simulink model "PeakDetect"  (R2018b)
settings: Solver=FixedStepAuto  StartTime=1  StopTime=20  FixedStep=1  RelTol=1e-3
libraries: hdlsllib x4, simulink x2
settings Model: FPTRunName=FPA_Reference  Creator=jason  LastModifiedBy=jason
settings OptimizationCC: DefaultParameterBehavior=Inlined

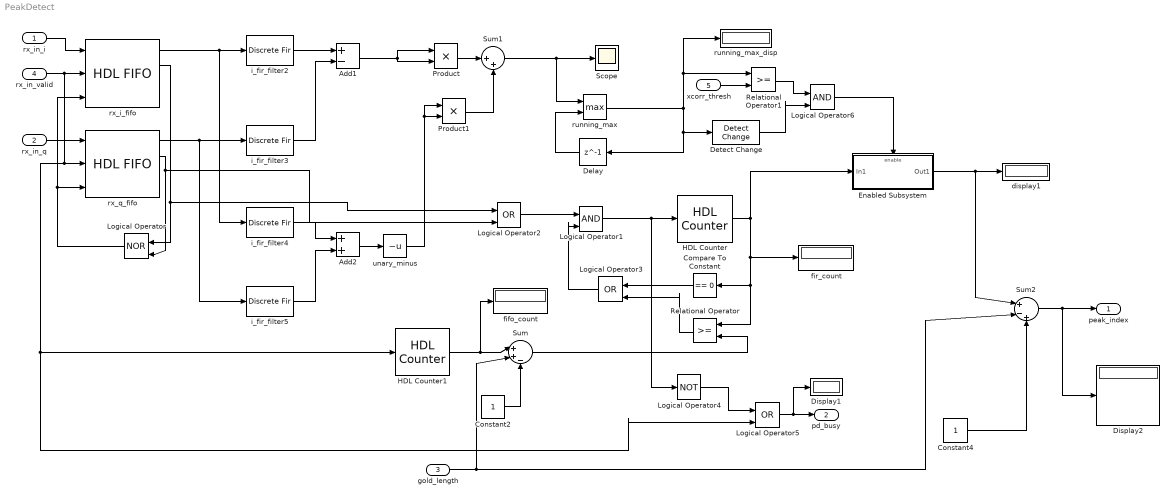
== system PeakDetect ==
  rx_in_i : Inport  OutDataTypeStr=fixdt(1,16,15)  SampleTime=1  Interpolate=off
  rx_in_q : Inport  Port=2  OutDataTypeStr=fixdt(1,16,15)  SampleTime=1  Interpolate=off
  gold_length : Inport  Port=3  OutDataTypeStr=uint16  Interpolate=off
  rx_in_valid : Inport  Port=4  OutDataTypeStr=boolean  SampleTime=1  Interpolate=off
  xcorr_thresh : Inport  Port=5  Interpolate=off
  Add1 : Sum  Inputs=+-
  Add2 : Sum
  Compare To Constant : simulink/Logic and Bit Operations/Compare To Constant  relop===  const=0  OutDataTypeStr=boolean
  Constant2 : Constant  OutDataTypeStr=uint8  SampleTime=-1
  Constant4 : Constant  OutDataTypeStr=uint16  SampleTime=-1
  Delay : Delay  DelayLength=1
  Detect Change : simulink/Logic and Bit Operations/Detect Change  vinit=0  OutDataTypeStr=boolean
  Display1 : Display
  Display2 : Display
  Enabled Subsystem : Subsystem  TreatAsAtomicUnit=on
  HDL Counter : hdlsllib/Sources/HDL Counter  CountType=Free running  CountInit=0  CountStep=1  CountMax=25  CountFromType=Initial value  CountFrom=0  CountResetPort=on  CountLoadPort=off  CountEnbPort=off  CountDirPort=off  CountDataType=Unsigned  CountWordLen=16  CountFracLen=0  CountSampTime=1
      settings: SourceProductBaseCode=HD
  HDL Counter1 : hdlsllib/Sources/HDL Counter  CountType=Free running  CountInit=0  CountStep=1  CountMax=25  CountFromType=Initial value  CountFrom=0  CountResetPort=off  CountLoadPort=off  CountEnbPort=on  CountDirPort=off  CountDataType=Unsigned  CountWordLen=16  CountFracLen=0  CountSampTime=1
      settings: SourceProductBaseCode=HD
  Logical Operator : Logic  Operator=NOR  IconShape=distinctive  AllPortsSameDT=off  OutDataTypeStr=boolean
  Logical Operator1 : Logic  IconShape=distinctive  AllPortsSameDT=off  OutDataTypeStr=boolean
  Logical Operator2 : Logic  Operator=OR  IconShape=distinctive  AllPortsSameDT=off  OutDataTypeStr=boolean
  Logical Operator3 : Logic  Operator=OR  IconShape=distinctive  AllPortsSameDT=off  OutDataTypeStr=boolean
  Logical Operator4 : Logic  Operator=NOT  IconShape=distinctive  AllPortsSameDT=off  OutDataTypeStr=boolean
  Logical Operator5 : Logic  Operator=OR  IconShape=distinctive  AllPortsSameDT=off  OutDataTypeStr=boolean
  Logical Operator6 : Logic  IconShape=distinctive  AllPortsSameDT=off  OutDataTypeStr=boolean
  Product : Product  OutDataTypeStr=Inherit: Inherit via back propagation
  Product1 : Product  OutDataTypeStr=Inherit: Inherit via back propagation
  Relational Operator : RelationalOperator  OutDataTypeStr=boolean  RndMeth=Nearest
  Relational Operator1 : RelationalOperator  OutDataTypeStr=boolean  RndMeth=Nearest
  Scope : Scope
  Sum : Sum  Inputs=|++-  AccumDataTypeStr=uint16
  Sum1 : Sum  Inputs=|++
  Sum2 : Sum  Inputs=|+-+  AccumDataTypeStr=uint16
  display1 : Display
  fifo_count : Display
  fir_count : Display
  i_fir_filter2 : DiscreteFir  Coefficients=fliplr([0.1538; 0.2282; 0.2753; 0.2904; 0.2678; 0.2226; 0.1475; 0.0555; -0.0424; -0.1347; -0.2101; -0.2594; -0.2722; -0.2594; -0.2101; -0.1347; -0.0424; 0.0555; 0.1475; 0.2226; 0.2763; 0.2977; 0.2794; 0.2276; 0.1477; 0.0478; -0.0623; -0.1725; -0.2689; -0.3564; -0.4163; -0.4493; -0.4546; -0.4329; -0.3872; -0.3214; -0.2364; -0.1508; -0.0581; 0.0313; 0.1114; 0.1768; 0.2233; 0.2478; 0.2445; 0.2267; 0.1835; 0.1230; 0.0499; -0.0298; -0.1101; -0.1852; -0.2545; -0.3086; -0.3404; -0.3536; -0.3500; -0.3325; -0.3055; -0.2736; -0.2459; -0.2136; -0.1926; -0.1807; -0.1788; -0.1865; -0.2027; -0.2254; -0.2478; -0.2799; -0.3056; -0.3262; -0.3387; -0.3401; -0.3282; -0.3015; -0.2637; -0.2106; -0.1396; -0.0592; 0.0251; 0.1067; 0.1795; 0.2379; 0.2826; 0.3069; 0.3069; 0.2909; 0.2651; 0.2369; 0.2138; 0.2018; 0.2005; 0.2156; 0.2494; 0.2914; 0.3326; 0.3631; 0.3737; 0.3572]')  ProductDataTypeStr=fixdt(1,64,32)  AccumDataTypeStr=fixdt(1,64,32)  OutDataTypeStr=fixdt(1,64,32)
  i_fir_filter3 : DiscreteFir  Coefficients=-1*fliplr([0.1538; 0.2282; 0.2753; 0.2904; 0.2678; 0.2226; 0.1475; 0.0555; -0.0424; -0.1347; -0.2101; -0.2594; -0.2722; -0.2594; -0.2101; -0.1347; -0.0424; 0.0555; 0.1475; 0.2226; 0.2763; 0.2977; 0.2794; 0.2276; 0.1477; 0.0478; -0.0623; -0.1725; -0.2689; -0.3564; -0.4163; -0.4493; -0.4546; -0.4329; -0.3872; -0.3214; -0.2364; -0.1508; -0.0581; 0.0313; 0.1114; 0.1768; 0.2233; 0.2478; 0.2445; 0.2267; 0.1835; 0.1230; 0.0499; -0.0298; -0.1101; -0.1852; -0.2545; -0.3086; -0.3404; -0.3536; -0.3500; -0.3325; -0.3055; -0.2736; -0.2459; -0.2136; -0.1926; -0.1807; -0.1788; -0.1865; -0.2027; -0.2254; -0.2478; -0.2799; -0.3056; -0.3262; -0.3387; -0.3401; -0.3282; -0.3015; -0.2637; -0.2106; -0.1396; -0.0592; 0.0251; 0.1067; 0.1795; 0.2379; 0.2826; 0.3069; 0.3069; 0.2909; 0.2651; 0.2369; 0.2138; 0.2018; 0.2005; 0.2156; 0.2494; 0.2914; 0.3326; 0.3631; 0.3737; 0.3572]')  ProductDataTypeStr=fixdt(1,64,32)  AccumDataTypeStr=fixdt(1,64,32)  OutDataTypeStr=fixdt(1,64,32)
  i_fir_filter4 : DiscreteFir  Coefficients=-1*fliplr([0.1538; 0.2282; 0.2753; 0.2904; 0.2678; 0.2226; 0.1475; 0.0555; -0.0424; -0.1347; -0.2101; -0.2594; -0.2722; -0.2594; -0.2101; -0.1347; -0.0424; 0.0555; 0.1475; 0.2226; 0.2763; 0.2977; 0.2794; 0.2276; 0.1477; 0.0478; -0.0623; -0.1725; -0.2689; -0.3564; -0.4163; -0.4493; -0.4546; -0.4329; -0.3872; -0.3214; -0.2364; -0.1508; -0.0581; 0.0313; 0.1114; 0.1768; 0.2233; 0.2478; 0.2445; 0.2267; 0.1835; 0.1230; 0.0499; -0.0298; -0.1101; -0.1852; -0.2545; -0.3086; -0.3404; -0.3536; -0.3500; -0.3325; -0.3055; -0.2736; -0.2459; -0.2136; -0.1926; -0.1807; -0.1788; -0.1865; -0.2027; -0.2254; -0.2478; -0.2799; -0.3056; -0.3262; -0.3387; -0.3401; -0.3282; -0.3015; -0.2637; -0.2106; -0.1396; -0.0592; 0.0251; 0.1067; 0.1795; 0.2379; 0.2826; 0.3069; 0.3069; 0.2909; 0.2651; 0.2369; 0.2138; 0.2018; 0.2005; 0.2156; 0.2494; 0.2914; 0.3326; 0.3631; 0.3737; 0.3572]')  ProductDataTypeStr=fixdt(1,64,32)  AccumDataTypeStr=fixdt(1,64,32)  OutDataTypeStr=fixdt(1,64,32)
  i_fir_filter5 : DiscreteFir  Coefficients=fliplr([0.1538; 0.2282; 0.2753; 0.2904; 0.2678; 0.2226; 0.1475; 0.0555; -0.0424; -0.1347; -0.2101; -0.2594; -0.2722; -0.2594; -0.2101; -0.1347; -0.0424; 0.0555; 0.1475; 0.2226; 0.2763; 0.2977; 0.2794; 0.2276; 0.1477; 0.0478; -0.0623; -0.1725; -0.2689; -0.3564; -0.4163; -0.4493; -0.4546; -0.4329; -0.3872; -0.3214; -0.2364; -0.1508; -0.0581; 0.0313; 0.1114; 0.1768; 0.2233; 0.2478; 0.2445; 0.2267; 0.1835; 0.1230; 0.0499; -0.0298; -0.1101; -0.1852; -0.2545; -0.3086; -0.3404; -0.3536; -0.3500; -0.3325; -0.3055; -0.2736; -0.2459; -0.2136; -0.1926; -0.1807; -0.1788; -0.1865; -0.2027; -0.2254; -0.2478; -0.2799; -0.3056; -0.3262; -0.3387; -0.3401; -0.3282; -0.3015; -0.2637; -0.2106; -0.1396; -0.0592; 0.0251; 0.1067; 0.1795; 0.2379; 0.2826; 0.3069; 0.3069; 0.2909; 0.2651; 0.2369; 0.2138; 0.2018; 0.2005; 0.2156; 0.2494; 0.2914; 0.3326; 0.3631; 0.3737; 0.3572]')  ProductDataTypeStr=fixdt(1,64,32)  AccumDataTypeStr=fixdt(1,64,32)  OutDataTypeStr=fixdt(1,64,32)
  running_max : MinMax  Function=max  Inputs=2
  running_max_disp : Display
  rx_i_fifo : hdlsllib/HDL RAMs/HDL FIFO  fifo_size=1024  ratio=1  push_msg=Warning  pop_msg=Warning  show_empty=on  show_full=on  show_num=on
      settings: SourceProductName=HDL Coder  SourceProductBaseCode=HD
  rx_q_fifo : hdlsllib/HDL RAMs/HDL FIFO  fifo_size=1024  ratio=1  push_msg=Warning  pop_msg=Warning  show_empty=on  show_full=on  show_num=on
      settings: SourceProductName=HDL Coder  SourceProductBaseCode=HD
  unary_minus : UnaryMinus
  peak_index : Outport  OutDataTypeStr=uint16
  pd_busy : Outport  Port=2
  wires:
  rx_in_i/1 -> rx_i_fifo/1
  Sum1/1 -> Scope/1, running_max/1
  i_fir_filter2/1 -> Add1/1
  i_fir_filter3/1 -> Add1/2
  i_fir_filter4/1 -> Add2/1
  i_fir_filter5/1 -> Add2/2
  Add1/1 -> Product/1, Product/2
  Add2/1 -> unary_minus/1
  Enabled Subsystem/1(Out1) -> display1/1, Sum2/1
  gold_length/1 -> Sum2/2, Sum/2
  Sum2/1 -> Display2/1, peak_index/1
  running_max/1 -> Detect Change/1, Delay/1, Relational Operator1/1, running_max_disp/1
  Delay/1 -> running_max/2
  rx_i_fifo/1 -> i_fir_filter4/1, i_fir_filter2/1
  rx_in_q/1 -> rx_q_fifo/1
  rx_q_fifo/1 -> i_fir_filter5/1, i_fir_filter3/1
  rx_in_valid/1 -> rx_q_fifo/2, Logical Operator5/2, HDL Counter1/1, rx_i_fifo/2
  rx_i_fifo/2 -> Logical Operator/1, Logical Operator2/1
  rx_q_fifo/2 -> Logical Operator/2, Logical Operator2/2
  Logical Operator/1 -> rx_q_fifo/3, rx_i_fifo/3
  Sum/1 -> Relational Operator/2
  Logical Operator1/1 -> Logical Operator4/1, HDL Counter/1
  Logical Operator2/1 -> Logical Operator1/1
  Compare To Constant/1 -> Logical Operator3/1
  Relational Operator/1 -> Logical Operator3/2
  Logical Operator3/1 -> Logical Operator1/2
  HDL Counter1/1 -> fifo_count/1, Sum/1
  HDL Counter/1 -> Compare To Constant/1, Relational Operator/1, fir_count/1, Enabled Subsystem/1(In1)
  Constant2/1 -> Sum/3
  Constant4/1 -> Sum2/3
  Logical Operator4/1 -> Logical Operator5/1
  Logical Operator5/1 -> Display1/1, pd_busy/1
  unary_minus/1 -> Product1/2, Product1/1
  Product/1 -> Sum1/1
  Product1/1 -> Sum1/2
  xcorr_thresh/1 -> Relational Operator1/2
  Relational Operator1/1 -> Logical Operator6/1
  Detect Change/1 -> Logical Operator6/2
  Logical Operator6/1 -> Enabled Subsystem/Enable

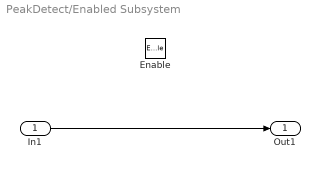
== system PeakDetect/Enabled Subsystem ==
  In1 : Inport
  Enable : EnablePort
  Out1 : Outport  InitialOutput=0
  wires:
  In1/1 -> Out1/1
